simulink model "P3"  (R2019a)
settings: Solver=VariableStepAuto  StartTime=0.0  StopTime=10.0  RelTol=1e-3
settings Model: Creator=john  LastModifiedBy=john

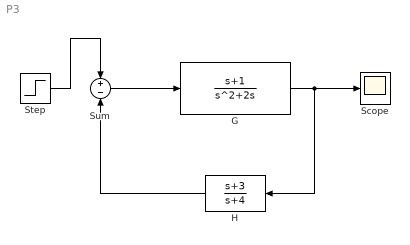
== system P3 ==
  G : TransferFcn  Numerator=[1 1]  Denominator=[1 2 0]
  H : TransferFcn  Numerator=[1 3]  Denominator=[1 4]
  Scope : Scope
  Step : Step  SampleTime=0
  Sum : Sum  Inputs=+-
  wires:
  G/1 -> Scope/1, H/1
  Sum/1 -> G/1
  Step/1 -> Sum/1
  H/1 -> Sum/2
